simulink model "assemblage_19"  (R2016a)
settings: Solver=ode15s  StartTime=0.0  StopTime=1e6  RelTol=1e-3
undefined symbols (not defined in the file or in its folder): W
libraries: simCryogenics_lib x424, nesl_utility x343, fl_lib x9
(part 1 of 3)
settings Model: Creator=bert  LastModifiedBy=FB229602
settings DataIOCC: LimitDataPoints=on  SaveFormat=Array
settings HardwareCC: ProdBitPerPointer=32  ProdLargestAtomicFloat=None  ProdIntDivRoundTo=Undefined  ProdEndianess=Unspecified  ProdWordSize=32  ProdHWDeviceType=32-bit Generic
settings ModelReferenceCC: PropagateSignalLabelsOutOfModel=off
settings ConfigComp: CovModelRefEnable=Off
settings SimscapeCC: SimscapeLogType=all

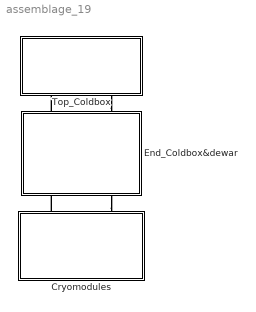
== system assemblage_19 ==
  Cryomodules : Subsystem
  End_Coldbox&dewar : Subsystem
  Top_Coldbox : Subsystem
  connections:
  End_Coldbox&dewar/RConn1 -- Top_Coldbox/LConn1
  Top_Coldbox/LConn2 -- End_Coldbox&dewar/RConn2
  End_Coldbox&dewar/LConn2 -- Cryomodules/RConn2
  Cryomodules/RConn1 -- End_Coldbox&dewar/LConn1

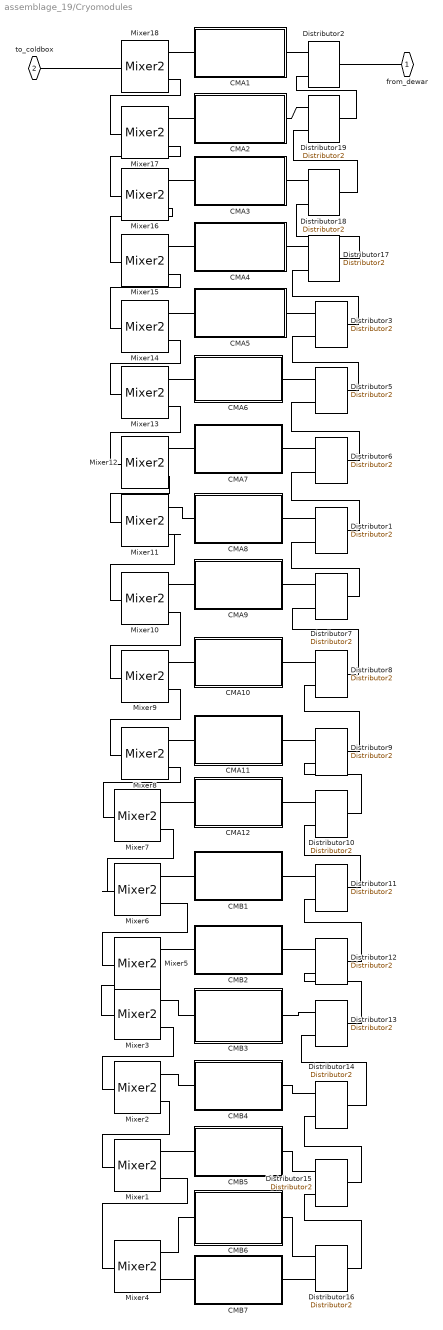
== system assemblage_19/Cryomodules ==
  CMA1 : Subsystem
  CMA10 : Subsystem
  CMA11 : Subsystem
  CMA12 : Subsystem
  CMA2 : Subsystem
  CMA3 : Subsystem
  CMA4 : Subsystem
  CMA5 : Subsystem
  CMA6 : Subsystem
  CMA7 : Subsystem
  CMA8 : Subsystem
  CMA9 : Subsystem
  CMB1 : Subsystem
  CMB2 : Subsystem
  CMB3 : Subsystem
  CMB4 : Subsystem
  CMB5 : Subsystem
  CMB6 : Subsystem
  CMB7 : Subsystem
  Distributor{1..3,5..19} (18 alike) : simCryogenics_lib/Elements/Distributor2
  Mixer{1..18} (18 alike) : simCryogenics_lib/Elements/Mixer2
  from_dewar : PMIOPort  Port=1  Side=Right
  to_coldbox : PMIOPort  Port=2  Side=Right
  connections:
  CMA1/RConn1 -- Distributor2/RConn2
  from_dewar/RConn1 -- Distributor2/LConn1
  Distributor1/RConn2 -- CMA8/RConn1
  CMA7/RConn1 -- Distributor6/RConn2
  CMA6/RConn1 -- Distributor5/RConn2
  CMA5/RConn1 -- Distributor3/RConn2
  Distributor3/RConn1 -- Distributor5/LConn1
  Distributor5/RConn1 -- Distributor6/LConn1
  Distributor6/RConn1 -- Distributor1/LConn1
  Distributor1/RConn1 -- Distributor7/LConn1
  Distributor7/RConn1 -- Distributor8/LConn1
  Distributor8/RConn1 -- Distributor9/LConn1
  Distributor10/LConn1 -- Distributor9/RConn1
  Distributor11/LConn1 -- Distributor10/RConn1
  Distributor11/RConn2 -- CMB1/RConn1
  Distributor10/RConn2 -- CMA12/RConn1
  Distributor9/RConn2 -- CMA11/RConn1
  CMA10/RConn1 -- Distributor8/RConn2
  CMA9/RConn1 -- Distributor7/RConn2
  Distributor12/LConn1 -- Distributor11/RConn1
  Distributor12/RConn2 -- CMB2/RConn1
  Distributor13/LConn1 -- Distributor12/RConn1
  Distributor13/RConn2 -- CMB3/RConn1
  Distributor14/LConn1 -- Distributor13/RConn1
  Distributor14/RConn2 -- CMB4/RConn1
  Distributor15/LConn1 -- Distributor14/RConn1
  Distributor15/RConn2 -- CMB5/RConn1
  Distributor16/LConn1 -- Distributor15/RConn1
  Distributor16/RConn2 -- CMB6/RConn1
  Distributor16/RConn1 -- CMB7/RConn1
  Distributor3/LConn1 -- Distributor17/RConn1
  Distributor17/RConn2 -- CMA4/RConn1
  Distributor18/RConn1 -- Distributor17/LConn1
  Distributor18/RConn2 -- CMA3/RConn1
  Distributor18/LConn1 -- Distributor19/RConn1
  Distributor19/RConn2 -- CMA2/RConn1
  Distributor2/RConn1 -- Distributor19/LConn1
  Mixer4/LConn1 -- CMB7/LConn1
  CMB6/LConn1 -- Mixer4/LConn2
  Mixer4/RConn1 -- Mixer1/LConn1
  CMB5/LConn1 -- Mixer1/LConn2
  Mixer2/LConn2 -- CMB4/LConn1
  Mixer1/RConn1 -- Mixer2/LConn1
  Mixer2/RConn1 -- Mixer3/LConn1
  CMB3/LConn1 -- Mixer3/LConn2
  Mixer5/LConn2 -- CMB2/LConn1
  Mixer3/RConn1 -- Mixer5/LConn1
  Mixer5/RConn1 -- Mixer6/LConn1
  Mixer6/LConn2 -- CMB1/LConn1
  Mixer6/RConn1 -- Mixer7/LConn1
  Mixer7/LConn2 -- CMA12/LConn1
  Mixer8/LConn1 -- Mixer7/RConn1
  Mixer8/LConn2 -- CMA11/LConn1
  Mixer9/LConn2 -- CMA10/LConn1
  Mixer9/LConn1 -- Mixer8/RConn1
  Mixer10/LConn2 -- CMA9/LConn1
  Mixer10/LConn1 -- Mixer9/RConn1
  Mixer11/LConn2 -- CMA8/LConn1
  Mixer11/LConn1 -- Mixer10/RConn1
  Mixer11/RConn1 -- Mixer12/LConn1
  Mixer12/LConn2 -- CMA7/LConn1
  Mixer13/LConn1 -- Mixer12/RConn1
  Mixer13/LConn2 -- CMA6/LConn1
  Mixer14/LConn1 -- Mixer13/RConn1
  Mixer14/LConn2 -- CMA5/LConn1
  Mixer15/LConn2 -- CMA4/LConn1
  Mixer15/LConn1 -- Mixer14/RConn1
  Mixer16/LConn2 -- CMA3/LConn1
  Mixer15/RConn1 -- Mixer16/LConn1
  Mixer17/LConn2 -- CMA2/LConn1
  Mixer18/LConn2 -- CMA1/LConn1
  Mixer17/LConn1 -- Mixer16/RConn1
  Mixer18/LConn1 -- Mixer17/RConn1
  Mixer18/RConn1 -- to_coldbox/RConn1

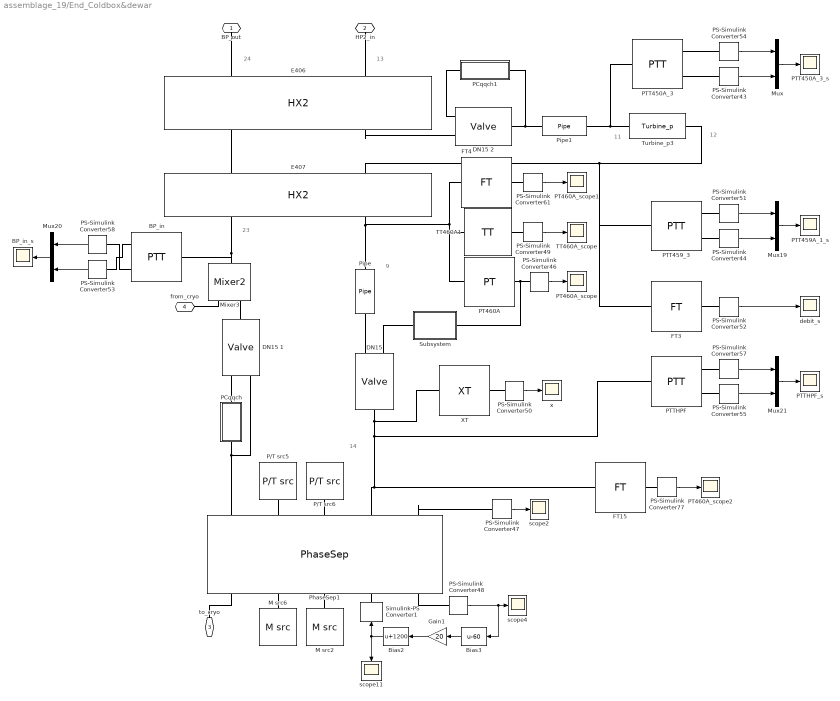
== system assemblage_19/End_Coldbox&dewar ==
  note: 13
  note: 24
  note: 9
  note: 14
  note: 11
  note: 12
  note: 23
  BP_in : simCryogenics_lib/Sensors/PTT
  "BP_in_s " : Scope
  Bias2 : Bias  Bias=1200
  Bias3 : Bias  Bias=-60
  "DN15 " : simCryogenics_lib/Elements/Valve  CVmax=1.5  ControlInputMin=0  ControlInputMax=100  Xt=0.86  Rv=10  lin_v=0  lim_v=0  K=2.4e-5 m^1.50000*kg^0.50000/s/bar^0.50000  Cmd_specify=off  Cmd_priority=High  Cmd=0  gamma_specify=off  gamma_priority=High  gamma=0  rho_specify=off  rho_priority=High  rho=0 kg/m^3  Xc_specify=off  Xc_priority=High  Xc=0  X_specify=off  X_priority=High  X=0  Y_specify=off  Y_priority=High  Y=0  CV_specify=off  CV_priority=High  CV=0
  DN15 1 : simCryogenics_lib/Elements/Valve  CVmax=40  ControlInputMin=0  ControlInputMax=100  Xt=0.86  Rv=50  lin_v=0  lim_v=0  K=2.4e-5 m^1.50000*kg^0.50000/s/bar^0.50000  Cmd_specify=off  Cmd_priority=High  Cmd=0  gamma_specify=off  gamma_priority=High  gamma=0  rho_specify=off  rho_priority=High  rho=0 kg/m^3  Xc_specify=off  Xc_priority=High  Xc=0  X_specify=off  X_priority=High  X=0  Y_specify=off  Y_priority=High  Y=0  CV_specify=off  CV_priority=High  CV=0
  DN15 2 : simCryogenics_lib/Elements/Valve  CVmax=4  ControlInputMin=0  ControlInputMax=100  Xt=0.86  Rv=50  lin_v=0  lim_v=0  K=2.4e-5 m^1.50000*kg^0.50000/s/bar^0.50000  Cmd_specify=off  Cmd_priority=High  Cmd=0  gamma_specify=off  gamma_priority=High  gamma=0  rho_specify=off  rho_priority=High  rho=0 kg/m^3  Xc_specify=off  Xc_priority=High  Xc=0  X_specify=off  X_priority=High  X=0  Y_specify=off  Y_priority=High  Y=0  CV_specify=off  CV_priority=High  CV=0
  E406 : simCryogenics_lib/Elements/HX2  N=9  Vh=0.065 m^3  Vc=0.023 m^3  M=64 kg  Kh=0.001/0.06439 s*bar/kg  Kc=0.0023/0.06368 s*bar/kg  h=1000 J/s/K  Th0=17 K  Ph0=14.73 bar  Mh0=0.06368 kg/s  Tc0=5 K  Pc0=1.05 bar  Mc0=0.06439 kg/s
  E407 : simCryogenics_lib/Elements/HX2  N=9  Vh=0.011 m^3  Vc=0.065 m^3  M=64 kg  Kh=0.002/0.06368 s*bar/kg  Kc=0.0023/0.06368 s*bar/kg  h=2000 J/s/K  Th0=5.7 K  Ph0=3.03 bar  Mh0=0.06368 kg/s  Tc0=4.4 K  Pc0=1.05 bar  Mc0=0.06368 kg/s
  FT15 : simCryogenics_lib/Sensors/FT
  FT3 : simCryogenics_lib/Sensors/FT
  FT4 : simCryogenics_lib/Sensors/FT
  Gain1 : Gain  Gain=20
  M src2 : simCryogenics_lib/Sources_Sinks/M src  M=0 kg/s
  M src6 : simCryogenics_lib/Sources_Sinks/M src  M=0 kg/s
  Mixer3 : simCryogenics_lib/Elements/Mixer2
  Mux{,19..21} (4 alike) : Mux  Inputs=2
  P/T src5 : simCryogenics_lib/Sources_Sinks/P//T src  P=5 bar  T=46.3 K
  P/T src6 : simCryogenics_lib/Sources_Sinks/P//T src  P=5 bar  T=46.3 K
  PCqqch : Subsystem
  PCqqch1 : Subsystem
  PS-Simulink Converter{43..44,46..55,57..58,61,77} (16 alike) : nesl_utility/PS-Simulink Converter  PhysicalDomain=network_engine_domain  SubClassName=ps_output  LeftPortType=input  RightPortType=output  PseudoPeriodic=off  Frequencies=[]  Unit=1  AffineConversion=off
  PT460A : simCryogenics_lib/Sensors/PT
  PT460A_scope : Scope
  PT460A_scope1 : Scope
  PT460A_scope2 : Scope
  PTT450A_3 : simCryogenics_lib/Sensors/PTT
  PTT450A_3_s : Scope
  PTT459A_1_s : Scope
  PTT459_3 : simCryogenics_lib/Sensors/PTT
  PTTHPF : simCryogenics_lib/Sensors/PTT
  PTTHPF_s : Scope
  PhaseSep1 : simCryogenics_lib/Elements/PhaseSep  Ideal1=1  DeltaT1=0.05 K  N1=10  h1=400 W/K  Ideal2=1  DeltaT2=0.05 K  N2=10  h2=400 W/K  hmax=1.601 m  S=3.4636 m^2  P0=1.3 atm  h0=20  T0=4.5 K
  Pipe : simCryogenics_lib/Elements/Pipe  Vol=0.01 m^3  Ideal=0  P0=3 bar  T0=4.6 K
  Pipe1 : simCryogenics_lib/Elements/Pipe  Vol=0.01 m^3  Ideal=0  P0=11 bar  T0=7.19 K
  Simulink-PS Converter1 : nesl_utility/Simulink-PS Converter  PhysicalDomain=network_engine_domain  SubClassName=ps_input  LeftPortType=input  RightPortType=output  PseudoPeriodic=off  Frequencies=[]  NoiseDistribution=none  NoiseParameters=[]  Unit=1  AffineConversion=off  InputFiltering=off  SimscapeFilterOrder=1  InputFilterTimeConstant=0.001  UdotUserProvided=1
  Subsystem : Subsystem
  TT460A1 : simCryogenics_lib/Sensors/TT
  TT460A_scope : Scope
  Turbine_p3 : simCryogenics_lib/Elements/Turbine_p  A=6.0851e-06 m^2  D=0.01 m  Mass=0.02 kg  cst_eff=1  eta0=0.75  Tin0=7.19 K  Pin0=14.73 bar  Pout0=3.03 bar  N0=2250 1/s  Q0=0 W  v0=0  I=0 kg*m^2  gamma_specify=off  gamma_priority=High  gamma=0  C_specify=off  C_priority=High  C=0  Z_specify=off  Z_priority=High  Z=0  Cp_specify=off  Cp_priority=High  Cp=0 kJ/kg/K  Sin_specify=off  Sin_priority=High  Sin=0 kJ/kg  T_specify=off  T_priority=High  T=0 K  HoutIs_specify=off  HoutIs_priority=High  HoutIs=0 kJ/kg  u1_specify=off  u1_priority=High  u1=0 m/s  c1_specify=off  c1_priority=High  c1=0 m/s  v_specify=off  v_priority=High  v=0  eta_specify=off  eta_priority=High  eta=0  eta_var_specify=off  eta_var_priority=High  eta_var=0  N_specify=off  N_priority=High  N=0 rad/s  Q_specify=off  Q_priority=High  Q=0 W
  XT : simCryogenics_lib/Sensors/XT
  debit_s : Scope
  scope11 : Scope
  scope2 : Scope
  scope4 : Scope
  x : Scope
  BP_out : PMIOPort  Port=1  Side=Right
  HP2_in : PMIOPort  Port=2  Side=Right
  to_cryo : PMIOPort  Port=3  Side=Left
  from_cryo : PMIOPort  Port=4  Side=Left
  wires:
  PS-Simulink Converter52/1 -> debit_s/1
  PS-Simulink Converter46/1 -> PT460A_scope/1
  PS-Simulink Converter49/1 -> TT460A_scope/1
  PS-Simulink Converter50/1 -> x/1
  PS-Simulink Converter54/1 -> Mux/1
  PS-Simulink Converter43/1 -> Mux/2
  Mux/1 -> PTT450A_3_s/1
  PS-Simulink Converter51/1 -> Mux19/1
  PS-Simulink Converter44/1 -> Mux19/2
  Mux19/1 -> PTT459A_1_s/1
  PS-Simulink Converter57/1 -> Mux21/1
  PS-Simulink Converter55/1 -> Mux21/2
  Mux21/1 -> PTTHPF_s/1
  Mux20/1 -> "BP_in_s "/1
  PS-Simulink Converter58/1 -> Mux20/1
  PS-Simulink Converter53/1 -> Mux20/2
  PS-Simulink Converter47/1 -> scope2/1
  PS-Simulink Converter61/1 -> PT460A_scope1/1
  PS-Simulink Converter77/1 -> PT460A_scope2/1
  Bias2/1 -> scope11/1, Simulink-PS Converter1/1
  PS-Simulink Converter48/1 -> Bias3/1, scope4/1
  Gain1/1 -> Bias2/1
  Bias3/1 -> Gain1/1
  connections:
  BP_in/LConn1 -- E407/RConn1 -- Mixer3/RConn1
  TT460A1/LConn1 -- PT460A/LConn1 -- FT4/LConn1 -- Pipe/LConn1 -- E407/RConn2
  E407/LConn2 -- PTT459_3/LConn1 -- FT3/LConn1 -- Turbine_p3/RConn1
  PhaseSep1/LConn4 -- FT15/LConn1 -- PTTHPF/LConn1 -- XT/LConn1 -- "DN15 "/RConn1
  PS-Simulink Converter46/LConn1 -- PT460A/RConn1 -- Subsystem/RConn1
  PhaseSep1/LConn5 -- PS-Simulink Converter47/LConn1
  BP_in/RConn1 -- PS-Simulink Converter58/LConn1
  PS-Simulink Converter50/LConn1 -- XT/RConn1
  M src2/RConn1 -- PhaseSep1/RConn3
  BP_in/RConn2 -- PS-Simulink Converter53/LConn1
  PhaseSep1/LConn2 -- P/T src5/RConn1
  E406/RConn1 -- E407/LConn1
  P/T src6/RConn1 -- PhaseSep1/LConn3
  PS-Simulink Converter44/LConn1 -- PTT459_3/RConn2
  PTT450A_3/RConn1 -- PS-Simulink Converter54/LConn1
  PS-Simulink Converter49/LConn1 -- TT460A1/RConn1
  PS-Simulink Converter55/LConn1 -- PTTHPF/RConn2
  PS-Simulink Converter52/LConn1 -- FT3/RConn1
  "DN15 "/LConn2 -- Pipe/RConn1
  M src6/RConn1 -- PhaseSep1/RConn2
  to_cryo/RConn1 -- PhaseSep1/RConn1
  PS-Simulink Converter51/LConn1 -- PTT459_3/RConn1
  PTT450A_3/RConn2 -- PS-Simulink Converter43/LConn1
  DN15 1/LConn2 -- PCqqch/LConn1 -- PhaseSep1/LConn1
  PTTHPF/RConn1 -- PS-Simulink Converter57/LConn1
  FT4/RConn1 -- PS-Simulink Converter61/LConn1
  Subsystem/LConn1 -- "DN15 "/LConn1
  FT15/RConn1 -- PS-Simulink Converter77/LConn1
  E406/LConn1 -- BP_out/RConn1
  HP2_in/RConn1 -- E406/LConn2
  PCqqch/RConn1 -- DN15 1/LConn1
  DN15 1/RConn1 -- Mixer3/LConn2
  from_cryo/RConn1 -- Mixer3/LConn1
  PCqqch1/RConn1 -- DN15 2/LConn1
  E406/RConn2 -- DN15 2/LConn2
  Turbine_p3/LConn1 -- Pipe1/RConn1 -- PTT450A_3/LConn1
  DN15 2/RConn1 -- Pipe1/LConn1 -- PCqqch1/LConn1
  PhaseSep1/RConn5 -- PS-Simulink Converter48/LConn1
  PhaseSep1/RConn4 -- Simulink-PS Converter1/RConn1

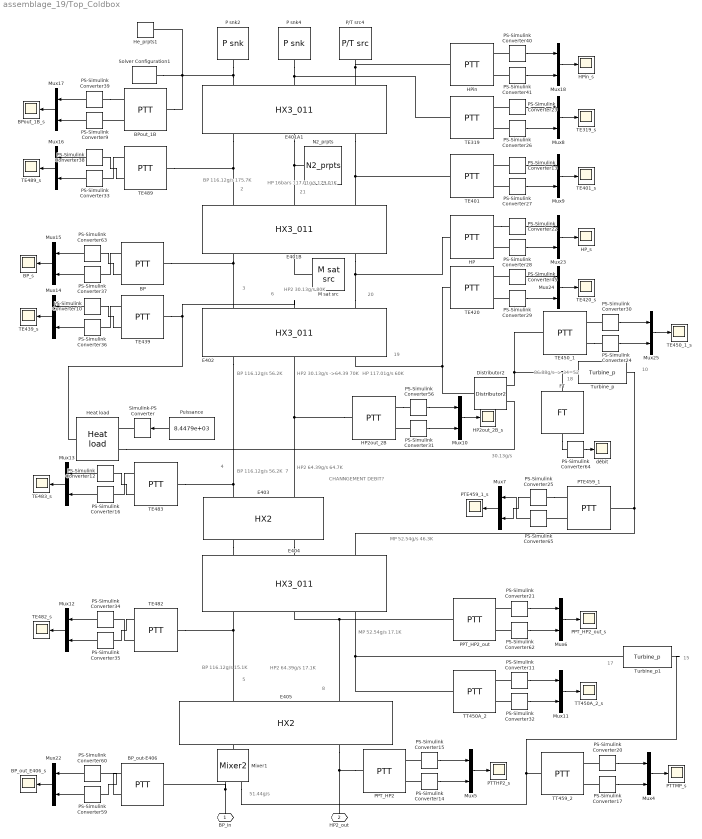
== system assemblage_19/Top_Coldbox ==
  note: 18
  note: 10
  note: 17
  note: 15
  note: 8
  note: 7
  note: 6
  note: 19
  note: 20
  note: 21
  note: 5
  note: 4
  note: 3
  note: 2
  note: HP
      | 16bars
      | 117.01g/s
      | 179.01K
  note: BP
      | 116.12g/s
      | 175.7K
  note: MP
      | 52.54g/s
      | 17.1K
  note: HP2
      | 64.39g/s
      | 17.1K
  note: BP
      | 116.12g/s
      | 15.1K
  note: MP
      | 52.54g/s
      | 46.3K
  note: CHANNGEMENT DEBIT?
  note: HP2
      | 64.39g/s
      | 64.7K
  note: BP
      | 116.12g/s
      | 56.2K
  note: 30.13g/s
  note: 86.88g/s
      | ->-34=52
  note: HP
      | 117.01g/s
      | 60K
  note: HP2
      | 30.13g/s ->64.39
      | 70K
  note: BP
      | 116.12g/s
      | 56.2K
  note: HP2
      | 30.13g/s
      | 80K
  note: 51.44g/s
  BP : simCryogenics_lib/Sensors/PTT
  BP_out-E406 : simCryogenics_lib/Sensors/PTT
  BP_out_E406_s : Scope
  BP_s : Scope
  BPout_1B : simCryogenics_lib/Sensors/PTT
  BPout_1B_s : Scope
  Distributor2 : simCryogenics_lib/Elements/Distributor2
  E401A1 : simCryogenics_lib/Elements/HX3_011  N=9  Vh=0.055 m^3  Vm=0.008 m^3  Vc=0.118 km^3  M=281 kg  Kh=0.033/0.11701 s*bar/kg  Km=0.021/.0026 s*bar/kg  Kc=0.062/0.11612 s*bar/kg  hh_m=2500 J/s/K  hh_c=1.8095e+04 J/s/K  hm_c=1 J/s/K  Th0=305 K  Ph0=14.73 bar  Mh0=0.11701 kg/s  Tm0=175.7 K  Pm0=1.1 bar  Mm0=0.0026 kg/s  Tc0=175.7 K  Pc0=1.05 bar  Mc0=0.11612 kg/s  sensh=0  sensm=1  sensc=1
  E401B : simCryogenics_lib/Elements/HX3_011  N=9  Vh=0.062 m^3  Vm=0.012 m^3  Vc=0.133 m^3  M=195 kg  Kh=0.017/0.11701 s*bar/kg  Km=0.002/(0.0026*4) s*bar/kg  Kc=0.051/0.11612 s*bar/kg  hh_m=7500 J/s/K  hh_c=25000 J/s/K  hm_c=1 J/s/K  Th0=179 K  Ph0=14.73 bar  Mh0=0.11701 kg/s  Tm0=80 K  Pm0=1.05 bar  Mm0=0.0026*4 kg/s  Tc0=80 K  Pc0=1.05 bar  Mc0=0.11612 kg/s  sensh=0  sensm=1  sensc=1
  E402 : simCryogenics_lib/Elements/HX3_011  N=9  Vh=0.133 m^3  Vm=0.005 m^3  Vc=0.012 m^3  M=195 kg  Kh=0.0255/0.11612 s*bar/kg  Km=0.011/0.03013 s*bar/kg  Kc=0.014/0.11701 s*bar/kg  hh_m=500 J/s/K  hh_c=3750 J/s/K  hm_c=1 J/s/K  Th0=56.2 K  Ph0=1.05 bar  Mh0=0.11612 kg/s  Tm0=80 K  Pm0=14.73 bar  Mm0=0.06439 kg/s  Tc0=100 K  Pc0=14.73 bar  Mc0=0.11701 kg/s  sensh=0  sensm=1  sensc=1
  E403 : simCryogenics_lib/Elements/HX2  N=9  Vh=0.049 m^3  Vc=0.172 m^3  M=227.5 kg  Kh=0.003/0.06439 s*bar/kg  Kc=0.0055/0.11612 s*bar/kg  h=5700 J/s/K  Th0=64.7 K  Ph0=14.73 bar  Mh0=0.116 kg/s  Tc0=46 K  Pc0=1.05 bar  Mc0=0.064 kg/s
  E404 : simCryogenics_lib/Elements/HX3_011  N=9  Vh=0.172 m^3  Vm=0.049 m^3  Vc=0.045 m^3  M=227.5 kg  Kh=0.0055/0.011612 s*bar/kg  Km=0.003/0.06439 s*bar/kg  Kc=0.004/0.05254 s*bar/kg  hh_m=11000 J/s/K  hh_c=8000 J/s/K  hm_c=1 J/s/K  Th0=15.1 K  Ph0=1.05 bar  Mh0=0.116 kg/s  Tm0=46 K  Pm0=14.73 bar  Mm0=0.064 kg/s  Tc0=46.3 K  Pc0=5 bar  Mc0=0.052 kg/s  sensh=0  sensm=1  sensc=1
  "E405 " : simCryogenics_lib/Elements/HX2  N=9  Vh=0.023 m^3  Vc=0.065 m^3  M=64 kg  Kh=0.001/0.6439 s*bar/kg  Kc=0.0023/0.11612 s*bar/kg  h=1500 J/s/K  Th0=17.1 K  Ph0=14.73 bar  Mh0=0.11612 kg/s  Tc0=10 K  Pc0=1.05 bar  Mc0=0.06439 kg/s
  FT : simCryogenics_lib/Sensors/FT
  HP : simCryogenics_lib/Sensors/PTT
  HP2out_2B : simCryogenics_lib/Sensors/PTT
  HP2out_2B_s : Scope
  HP_s : Scope
  HPin : simCryogenics_lib/Sensors/PTT
  HPin_s : Scope
  He_prpts1 : simCryogenics_lib/Utilities/He_prpts  P_min=0.1 bar  P_max=30 bar  T_min=3 K  T_max=320 K  N=100  Mol=4.0026 * 10 ^ (- 3) kg/mol
  Heat load : simCryogenics_lib/Utilities/Heat load
  M sat src : simCryogenics_lib/Sources_Sinks/M sat src  M=0.015 kg/s  Xmix=0
  Mixer1 : simCryogenics_lib/Elements/Mixer2
  Mux{4..18,22..25} (19 alike) : Mux  Inputs=2
  N2_prpts : simCryogenics_lib/Utilities/N2_prpts  P_min=0.5 bar  T_min=70 K  T_max=320 K  P_max=20 bar  Mol=4.0026 * (10 ^ (- 3)) kg/mol
  P snk2 : simCryogenics_lib/Sources_Sinks/P snk  P=1.05 bar
  P snk4 : simCryogenics_lib/Sources_Sinks/P snk  P=1.05 bar
  P/T src4 : simCryogenics_lib/Sources_Sinks/P//T src  P=14.73 bar  T=305 K
  PPT_HP2 : simCryogenics_lib/Sensors/PTT
  PPT_HP2_out : simCryogenics_lib/Sensors/PTT
  PPT_HP2_out_s : Scope
  PS-Simulink Converter{9..17,20..41,45,56,59..60,62..65} (39 alike) : nesl_utility/PS-Simulink Converter  PhysicalDomain=network_engine_domain  SubClassName=ps_output  LeftPortType=input  RightPortType=output  PseudoPeriodic=off  Frequencies=[]  Unit=1  AffineConversion=off
  PTE459_1 : simCryogenics_lib/Sensors/PTT
  PTE459_1_s : Scope
  PTTHP2_s : Scope
  PTTMP_s : Scope
  "Puissance " : Constant  Value=8.4479e+03
  Simulink-PS Converter : nesl_utility/Simulink-PS Converter  PhysicalDomain=network_engine_domain  SubClassName=ps_input  LeftPortType=input  RightPortType=output  PseudoPeriodic=off  Frequencies=[]  NoiseDistribution=none  NoiseParameters=[]  Unit=1  AffineConversion=off  InputFiltering=off  SimscapeFilterOrder=1  InputFilterTimeConstant=0.001  UdotUserProvided=1
  Solver Configuration1 : nesl_utility/Solver Configuration  PhysicalDomain=network_engine_domain  SubClassName=solver  LeftPortType=input  RightPortType=generic  Accelerate=off  Tones=[]  Harmonics=[]  SimulateNoise=off  Profile=off  UseLocalSampling=off  EnableSwitchedLinearOptims=on  FrequencyDomain=off  UseCCode=off  RelTol=0.001  AbsTol=1e-06  MinStep=1e-09  ToWorkspace=off  RevertToSquareIcSolve=off  NumHomotopyIterations=100  PhasorMode=off  PhasorModeNumHarmonics=1  OverrideAbsTol=off  DoDC=off  ResidualTolerance=1e-09  UseLocalSolver=off  LocalSolverChoice=NE_BACKWARD_EULER_ADVANCER  LocalSolverSampleTime=0.001  DoFixedCost=off  MaxNonlinIter=3  MaxModeIter=2  LinearAlgebra=Sparse  DelaysMemoryBudget=1024  AutomaticFiltering=on  FilteringTimeConstant=0.001
  TE{319,401,420,439,482..483,489} (7 alike) : simCryogenics_lib/Sensors/PTT
  TE319_s : Scope
  TE401_s : Scope
  TE420_s : Scope
  TE439_s : Scope
  TE450_1 : simCryogenics_lib/Sensors/PTT
  TE450_1_s : Scope
  TE482_s : Scope
  TE483_s : Scope
  TE489_s : Scope
  TT450A_2 : simCryogenics_lib/Sensors/PTT
  TT450A_2_s : Scope
  TT459_2 : simCryogenics_lib/Sensors/PTT
  Turbine_p : simCryogenics_lib/Elements/Turbine_p  A=1.7590e-05 m^2  D=0.035 m  Mass=0.02 kg  cst_eff=1  eta0=0.75  Tin0=80 K  Pin0=14.73 bar  Pout0=5.3 bar  N0=2250 1/s  Q0=0 W  v0=0  I=0 kg*m^2  gamma_specify=off  gamma_priority=High  gamma=0  C_specify=off  C_priority=High  C=0  Z_specify=off  Z_priority=High  Z=0  Cp_specify=off  Cp_priority=High  Cp=0 kJ/kg/K  Sin_specify=off  Sin_priority=High  Sin=0 kJ/kg  T_specify=off  T_priority=High  T=0 K  HoutIs_specify=off  HoutIs_priority=High  HoutIs=0 kJ/kg  u1_specify=off  u1_priority=High  u1=0 m/s  c1_specify=off  c1_priority=High  c1=0 m/s  v_specify=off  v_priority=High  v=0  eta_specify=off  eta_priority=High  eta=0  eta_var_specify=off  eta_var_priority=High  eta_var=0  N_specify=off  N_priority=High  N=0 rad/s  Q_specify=off  Q_priority=High  Q=0 W
  Turbine_p1 : simCryogenics_lib/Elements/Turbine_p  A=2.6523e-05 m^2  D=0.02 m  Mass=0.02 kg  cst_eff=1  eta0=0.75  Tin0=17.1 K  Pin0=5 bar  Pout0=1.3 bar  N0=2250 1/s  Q0=0 W  v0=0  I=0 kg*m^2  gamma_specify=off  gamma_priority=High  gamma=0  C_specify=off  C_priority=High  C=0  Z_specify=off  Z_priority=High  Z=0  Cp_specify=off  Cp_priority=High  Cp=0 kJ/kg/K  Sin_specify=off  Sin_priority=High  Sin=0 kJ/kg  T_specify=off  T_priority=High  T=0 K  HoutIs_specify=off  HoutIs_priority=High  HoutIs=0 kJ/kg  u1_specify=off  u1_priority=High  u1=0 m/s  c1_specify=off  c1_priority=High  c1=0 m/s  v_specify=off  v_priority=High  v=0  eta_specify=off  eta_priority=High  eta=0  eta_var_specify=off  eta_var_priority=High  eta_var=0  N_specify=off  N_priority=High  N=0 rad/s  Q_specify=off  Q_priority=High  Q=0 W
  débit : Scope
  BP_in : PMIOPort  Port=1  Side=Left
  HP2_out : PMIOPort  Port=2  Side=Left
  wires:
  "Puissance "/1 -> Simulink-PS Converter/1
  PS-Simulink Converter64/1 -> débit/1
  PS-Simulink Converter15/1 -> Mux5/1
  PS-Simulink Converter14/1 -> Mux5/2
  Mux5/1 -> PTTHP2_s/1
  PS-Simulink Converter20/1 -> Mux4/1
  PS-Simulink Converter17/1 -> Mux4/2
  Mux4/1 -> PTTMP_s/1
  PS-Simulink Converter21/1 -> Mux6/1
  PS-Simulink Converter62/1 -> Mux6/2
  Mux6/1 -> PPT_HP2_out_s/1
  Mux7/1 -> PTE459_1_s/1
  PS-Simulink Converter23/1 -> Mux8/1
  PS-Simulink Converter26/1 -> Mux8/2
  Mux8/1 -> TE319_s/1
  PS-Simulink Converter13/1 -> Mux9/1
  PS-Simulink Converter27/1 -> Mux9/2
  Mux9/1 -> TE401_s/1
  PS-Simulink Converter28/1 -> Mux23/2
  Mux23/1 -> HP_s/1
  PS-Simulink Converter45/1 -> Mux24/1
  PS-Simulink Converter29/1 -> Mux24/2
  Mux24/1 -> TE420_s/1
  PS-Simulink Converter30/1 -> Mux25/1
  Mux25/1 -> TE450_1_s/1
  PS-Simulink Converter22/1 -> Mux23/1
  PS-Simulink Converter31/1 -> Mux10/2
  Mux10/1 -> HP2out_2B_s/1
  PS-Simulink Converter56/1 -> Mux10/1
  PS-Simulink Converter11/1 -> Mux11/1
  PS-Simulink Converter32/1 -> Mux11/2
  Mux11/1 -> TT450A_2_s/1
  Mux12/1 -> TE482_s/1
  PS-Simulink Converter34/1 -> Mux12/1
  PS-Simulink Converter35/1 -> Mux12/2
  Mux13/1 -> TE483_s/1
  PS-Simulink Converter12/1 -> Mux13/1
  PS-Simulink Converter16/1 -> Mux13/2
  Mux14/1 -> TE439_s/1
  PS-Simulink Converter10/1 -> Mux14/1
  PS-Simulink Converter36/1 -> Mux14/2
  Mux15/1 -> BP_s/1
  PS-Simulink Converter63/1 -> Mux15/1
  PS-Simulink Converter37/1 -> Mux15/2
  Mux16/1 -> TE489_s/1
  PS-Simulink Converter38/1 -> Mux16/1
  PS-Simulink Converter33/1 -> Mux16/2
  Mux17/1 -> BPout_1B_s/1
  PS-Simulink Converter39/1 -> Mux17/1
  PS-Simulink Converter9/1 -> Mux17/2
  PS-Simulink Converter65/1 -> Mux7/1
  PS-Simulink Converter25/1 -> Mux7/2
  PS-Simulink Converter24/1 -> Mux25/2
  PS-Simulink Converter40/1 -> Mux18/1
  PS-Simulink Converter41/1 -> Mux18/2
  Mux18/1 -> HPin_s/1
  Mux22/1 -> BP_out_E406_s/1
  PS-Simulink Converter60/1 -> Mux22/1
  PS-Simulink Converter59/1 -> Mux22/2
  connections:
  TE482/LConn1 -- "E405 "/LConn1 -- E404/LConn3
  TE483/LConn1 -- E402/LConn3 -- E403/LConn1
  HP2out_2B/LConn1 -- E403/LConn2 -- E402/LConn2
  PPT_HP2_out/LConn1 -- "E405 "/LConn2 -- E404/LConn2
  Turbine_p1/LConn1 -- TT450A_2/LConn1 -- E404/LConn1
  PTE459_1/LConn1 -- Turbine_p/RConn1 -- E404/RConn1
  BP/LConn1 -- E401B/RConn1 -- E402/RConn3
  E401A1/RConn1 -- TE489/LConn1 -- E401B/LConn1
  E402/RConn1 -- HP/LConn1 -- E401B/RConn3
  E402/LConn1 -- Distributor2/LConn1 -- TE420/LConn1
  E402/RConn2 -- Heat load/RConn1 -- TE439/LConn1
  Turbine_p/LConn1 -- FT/LConn1 -- TE450_1/LConn1 -- Distributor2/RConn1
  Turbine_p1/RConn1 -- Mixer1/LConn2 -- TT459_2/LConn1
  E401A1/RConn3 -- E401B/LConn3 -- TE401/LConn1
  PPT_HP2/LConn1 -- "E405 "/RConn2 -- HP2_out/RConn1
  Mixer1/LConn1 -- BP_in/RConn1 -- BP_out-E406/LConn1
  HPin/LConn1 -- P/T src4/RConn1 -- E401A1/LConn3
  E401A1/LConn2 -- P snk4/RConn1 -- TE319/LConn1
  E401A1/LConn1 -- Solver Configuration1/RConn1 -- He_prpts1/RConn1 -- BPout_1B/LConn1 -- P snk2/RConn1
  PS-Simulink Converter38/LConn1 -- TE489/RConn1
  TE489/RConn2 -- PS-Simulink Converter33/LConn1
  BPout_1B/RConn2 -- PS-Simulink Converter9/LConn1
  PS-Simulink Converter39/LConn1 -- BPout_1B/RConn1
  PS-Simulink Converter40/LConn1 -- HPin/RConn1
  PS-Simulink Converter41/LConn1 -- HPin/RConn2
  BP_out-E406/RConn1 -- PS-Simulink Converter60/LConn1
  PS-Simulink Converter26/LConn1 -- TE319/RConn2
  E403/RConn2 -- E404/RConn2
  PS-Simulink Converter25/LConn1 -- PTE459_1/RConn2
  TE450_1/RConn2 -- PS-Simulink Converter24/LConn1
  PS-Simulink Converter62/LConn1 -- PPT_HP2_out/RConn2
  PS-Simulink Converter11/LConn1 -- TT450A_2/RConn1
  PS-Simulink Converter21/LConn1 -- PPT_HP2_out/RConn1
  PS-Simulink Converter20/LConn1 -- TT459_2/RConn1
  PS-Simulink Converter32/LConn1 -- TT450A_2/RConn2
  E401A1/RConn2 -- N2_prpts/RConn1 -- E401B/LConn2
  M sat src/RConn1 -- E401B/RConn2
  PS-Simulink Converter17/LConn1 -- TT459_2/RConn2
  PS-Simulink Converter31/LConn1 -- HP2out_2B/RConn2
  PS-Simulink Converter15/LConn1 -- PPT_HP2/RConn1
  HP2out_2B/RConn1 -- PS-Simulink Converter56/LConn1
  PS-Simulink Converter14/LConn1 -- PPT_HP2/RConn2
  Mixer1/RConn1 -- "E405 "/RConn1
  HP/RConn1 -- PS-Simulink Converter22/LConn1
  FT/RConn1 -- PS-Simulink Converter64/LConn1
  PS-Simulink Converter30/LConn1 -- TE450_1/RConn1
  PS-Simulink Converter29/LConn1 -- TE420/RConn2
  PS-Simulink Converter45/LConn1 -- TE420/RConn1
  Simulink-PS Converter/RConn1 -- Heat load/LConn2
  Heat load/LConn1 -- Distributor2/RConn2
  PS-Simulink Converter28/LConn1 -- HP/RConn2
  PS-Simulink Converter13/LConn1 -- TE401/RConn1
  PS-Simulink Converter27/LConn1 -- TE401/RConn2
  PTE459_1/RConn1 -- PS-Simulink Converter65/LConn1
  E403/RConn1 -- E404/RConn3
  BP_out-E406/RConn2 -- PS-Simulink Converter59/LConn1
  PS-Simulink Converter23/LConn1 -- TE319/RConn1
  TE483/RConn2 -- PS-Simulink Converter16/LConn1
  PS-Simulink Converter12/LConn1 -- TE483/RConn1
  TE482/RConn2 -- PS-Simulink Converter35/LConn1
  TE482/RConn1 -- PS-Simulink Converter34/LConn1
  TE439/RConn2 -- PS-Simulink Converter36/LConn1
  PS-Simulink Converter10/LConn1 -- TE439/RConn1
  BP/RConn2 -- PS-Simulink Converter37/LConn1
  PS-Simulink Converter63/LConn1 -- BP/RConn1

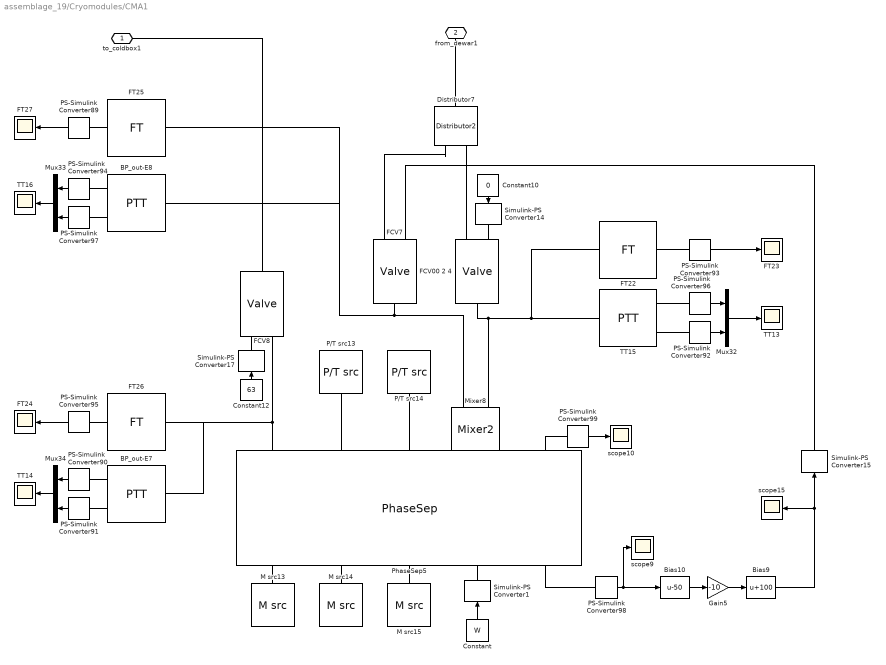
== system assemblage_19/Cryomodules/CMA1 ==
  BP_out-E7 : simCryogenics_lib/Sensors/PTT
  BP_out-E8 : simCryogenics_lib/Sensors/PTT
  Bias10 : Bias  Bias=-50
  Bias9 : Bias  Bias=100
  Constant : Constant  Value=W
  Constant10 : Constant  Value=0
  Constant12 : Constant  Value=63
  Distributor7 : simCryogenics_lib/Elements/Distributor2
  FCV00 2 4 : simCryogenics_lib/Elements/Valve  CVmax=0.2  ControlInputMin=0  ControlInputMax=100  Xt=0.86  Rv=100  lin_v=0  lim_v=0  K=2.4e-5 m^1.50000*kg^0.50000/s/bar^0.50000  Cmd_specify=off  Cmd_priority=High  Cmd=0  gamma_specify=off  gamma_priority=High  gamma=0  rho_specify=off  rho_priority=High  rho=0 kg/m^3  Xc_specify=off  Xc_priority=High  Xc=0  X_specify=off  X_priority=High  X=0  Y_specify=off  Y_priority=High  Y=0  CV_specify=off  CV_priority=High  CV=0
  FCV7 : simCryogenics_lib/Elements/Valve  CVmax=1.25  ControlInputMin=0  ControlInputMax=100  Xt=0.86  Rv=150  lin_v=0  lim_v=0  K=2.4e-5 m^1.50000*kg^0.50000/s/bar^0.50000  Cmd_specify=off  Cmd_priority=High  Cmd=0  gamma_specify=off  gamma_priority=High  gamma=0  rho_specify=off  rho_priority=High  rho=0 kg/m^3  Xc_specify=off  Xc_priority=High  Xc=0  X_specify=off  X_priority=High  X=0  Y_specify=off  Y_priority=High  Y=0  CV_specify=off  CV_priority=High  CV=0
  FCV8 : simCryogenics_lib/Elements/Valve  CVmax=1.5  ControlInputMin=0  ControlInputMax=100  Xt=0.86  Rv=100  lin_v=0  lim_v=0  K=2.4e-5 m^1.50000*kg^0.50000/s/bar^0.50000  Cmd_specify=off  Cmd_priority=High  Cmd=0  gamma_specify=off  gamma_priority=High  gamma=0  rho_specify=off  rho_priority=High  rho=0 kg/m^3  Xc_specify=off  Xc_priority=High  Xc=0  X_specify=off  X_priority=High  X=0  Y_specify=off  Y_priority=High  Y=0  CV_specify=off  CV_priority=High  CV=0
  FT22 : simCryogenics_lib/Sensors/FT
  FT23 : Scope
  FT24 : Scope
  FT25 : simCryogenics_lib/Sensors/FT
  FT26 : simCryogenics_lib/Sensors/FT
  FT27 : Scope
  Gain5 : Gain  Gain=-10
  M src13 : simCryogenics_lib/Sources_Sinks/M src  M=0 kg/s
  M src14 : simCryogenics_lib/Sources_Sinks/M src  M=0 kg/s
  M src15 : simCryogenics_lib/Sources_Sinks/M src  M=0 kg/s
  Mixer8 : simCryogenics_lib/Elements/Mixer2
  Mux32 : Mux  Inputs=2
  Mux33 : Mux  Inputs=2
  Mux34 : Mux  Inputs=2
  P/T src13 : simCryogenics_lib/Sources_Sinks/P//T src  P=1.2 bar  T=4.4 K
  P/T src14 : simCryogenics_lib/Sources_Sinks/P//T src  P=1.2 bar  T=4.4 K
  PS-Simulink Converter{89..99} (11 alike) : nesl_utility/PS-Simulink Converter  PhysicalDomain=network_engine_domain  SubClassName=ps_output  LeftPortType=input  RightPortType=output  PseudoPeriodic=off  Frequencies=[]  Unit=1  AffineConversion=off
  PhaseSep5 : simCryogenics_lib/Elements/PhaseSep  Ideal1=1  DeltaT1=0.05 K  N1=10  h1=400 W/K  Ideal2=1  DeltaT2=0.05 K  N2=10  h2=400 W/K  hmax=0.870 m  S=0.0402 m^2  P0=1.25 bar  h0=50  T0=4.5 K
  Simulink-PS Converter{1,14..15,17} (4 alike) : nesl_utility/Simulink-PS Converter  PhysicalDomain=network_engine_domain  SubClassName=ps_input  LeftPortType=input  RightPortType=output  PseudoPeriodic=off  Frequencies=[]  NoiseDistribution=none  NoiseParameters=[]  Unit=1  AffineConversion=off  InputFiltering=off  SimscapeFilterOrder=1  InputFilterTimeConstant=0.001  UdotUserProvided=1
  TT13 : Scope
  TT14 : Scope
  TT15 : simCryogenics_lib/Sensors/PTT
  TT16 : Scope
  scope10 : Scope
  scope15 : Scope
  scope9 : Scope
  to_coldbox1 : PMIOPort  Port=1  Side=Left
  from_dewar1 : PMIOPort  Port=2  Side=Right
  wires:
  Constant10/1 -> Simulink-PS Converter14/1
  PS-Simulink Converter99/1 -> scope10/1
  PS-Simulink Converter90/1 -> Mux34/1
  PS-Simulink Converter95/1 -> FT24/1
  Bias10/1 -> Gain5/1
  PS-Simulink Converter96/1 -> Mux32/1
  Constant/1 -> Simulink-PS Converter1/1
  Bias9/1 -> scope15/1, Simulink-PS Converter15/1
  Mux33/1 -> TT16/1
  PS-Simulink Converter89/1 -> FT27/1
  PS-Simulink Converter97/1 -> Mux33/2
  PS-Simulink Converter94/1 -> Mux33/1
  PS-Simulink Converter91/1 -> Mux34/2
  PS-Simulink Converter93/1 -> FT23/1
  Mux34/1 -> TT14/1
  PS-Simulink Converter92/1 -> Mux32/2
  Gain5/1 -> Bias9/1
  PS-Simulink Converter98/1 -> scope9/1, Bias10/1
  Mux32/1 -> TT13/1
  Constant12/1 -> Simulink-PS Converter17/1
  connections:
  BP_out-E8/RConn1 -- PS-Simulink Converter97/LConn1
  Simulink-PS Converter14/RConn1 -- FCV00 2 4/LConn1
  Distributor7/RConn2 -- FCV7/LConn2
  PS-Simulink Converter98/LConn1 -- PhaseSep5/RConn5
  from_dewar1/RConn1 -- Distributor7/LConn1
  TT15/RConn1 -- PS-Simulink Converter96/LConn1
  PhaseSep5/LConn2 -- P/T src13/RConn1
  FCV8/LConn2 -- PhaseSep5/LConn1 -- BP_out-E7/LConn1 -- FT26/LConn1
  FCV8/RConn1 -- to_coldbox1/RConn1
  P/T src14/RConn1 -- PhaseSep5/LConn3
  BP_out-E7/RConn2 -- PS-Simulink Converter90/LConn1
  FT22/LConn1 -- TT15/LConn1 -- FCV00 2 4/RConn1 -- Mixer8/LConn1
  FCV7/RConn1 -- Mixer8/LConn2 -- FT25/LConn1 -- BP_out-E8/LConn1
  Simulink-PS Converter15/RConn1 -- FCV7/LConn1
  M src15/RConn1 -- PhaseSep5/RConn3
  Simulink-PS Converter1/RConn1 -- PhaseSep5/RConn4
  BP_out-E7/RConn1 -- PS-Simulink Converter91/LConn1
  PS-Simulink Converter93/LConn1 -- FT22/RConn1
  BP_out-E8/RConn2 -- PS-Simulink Converter94/LConn1
  PhaseSep5/RConn2 -- M src14/RConn1
  PS-Simulink Converter89/LConn1 -- FT25/RConn1
  PS-Simulink Converter99/LConn1 -- PhaseSep5/LConn5
  TT15/RConn2 -- PS-Simulink Converter92/LConn1
  FCV00 2 4/LConn2 -- Distributor7/RConn1
  M src13/RConn1 -- PhaseSep5/RConn1
  PS-Simulink Converter95/LConn1 -- FT26/RConn1
  FCV8/LConn1 -- Simulink-PS Converter17/RConn1
  PhaseSep5/LConn4 -- Mixer8/RConn1

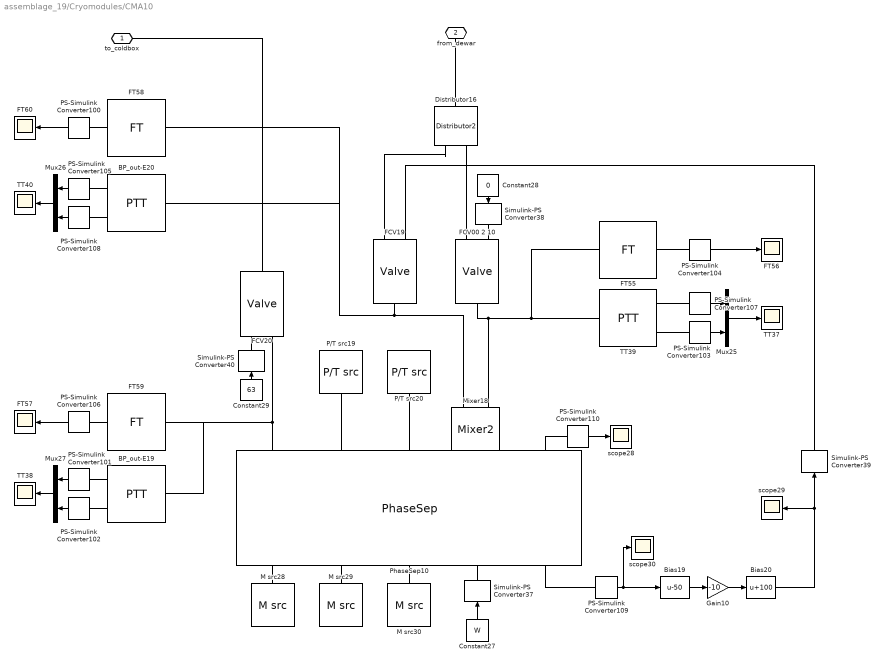
== system assemblage_19/Cryomodules/CMA10 ==
  BP_out-E19 : simCryogenics_lib/Sensors/PTT
  BP_out-E20 : simCryogenics_lib/Sensors/PTT
  Bias19 : Bias  Bias=-50
  Bias20 : Bias  Bias=100
  Constant27 : Constant  Value=W
  Constant28 : Constant  Value=0
  Constant29 : Constant  Value=63
  Distributor16 : simCryogenics_lib/Elements/Distributor2
  FCV00 2 10 : simCryogenics_lib/Elements/Valve  CVmax=0.2  ControlInputMin=0  ControlInputMax=100  Xt=0.86  Rv=100  lin_v=0  lim_v=0  K=2.4e-5 m^1.50000*kg^0.50000/s/bar^0.50000  Cmd_specify=off  Cmd_priority=High  Cmd=0  gamma_specify=off  gamma_priority=High  gamma=0  rho_specify=off  rho_priority=High  rho=0 kg/m^3  Xc_specify=off  Xc_priority=High  Xc=0  X_specify=off  X_priority=High  X=0  Y_specify=off  Y_priority=High  Y=0  CV_specify=off  CV_priority=High  CV=0
  FCV19 : simCryogenics_lib/Elements/Valve  CVmax=1.25  ControlInputMin=0  ControlInputMax=100  Xt=0.86  Rv=150  lin_v=0  lim_v=0  K=2.4e-5 m^1.50000*kg^0.50000/s/bar^0.50000  Cmd_specify=off  Cmd_priority=High  Cmd=0  gamma_specify=off  gamma_priority=High  gamma=0  rho_specify=off  rho_priority=High  rho=0 kg/m^3  Xc_specify=off  Xc_priority=High  Xc=0  X_specify=off  X_priority=High  X=0  Y_specify=off  Y_priority=High  Y=0  CV_specify=off  CV_priority=High  CV=0
  FCV20 : simCryogenics_lib/Elements/Valve  CVmax=1.5  ControlInputMin=0  ControlInputMax=100  Xt=0.86  Rv=100  lin_v=0  lim_v=0  K=2.4e-5 m^1.50000*kg^0.50000/s/bar^0.50000  Cmd_specify=off  Cmd_priority=High  Cmd=0  gamma_specify=off  gamma_priority=High  gamma=0  rho_specify=off  rho_priority=High  rho=0 kg/m^3  Xc_specify=off  Xc_priority=High  Xc=0  X_specify=off  X_priority=High  X=0  Y_specify=off  Y_priority=High  Y=0  CV_specify=off  CV_priority=High  CV=0
  FT55 : simCryogenics_lib/Sensors/FT
  FT56 : Scope
  FT57 : Scope
  FT58 : simCryogenics_lib/Sensors/FT
  FT59 : simCryogenics_lib/Sensors/FT
  FT60 : Scope
  Gain10 : Gain  Gain=-10
  M src28 : simCryogenics_lib/Sources_Sinks/M src  M=0 kg/s
  M src29 : simCryogenics_lib/Sources_Sinks/M src  M=0 kg/s
  M src30 : simCryogenics_lib/Sources_Sinks/M src  M=0 kg/s
  Mixer18 : simCryogenics_lib/Elements/Mixer2
  Mux25 : Mux  Inputs=2
  Mux26 : Mux  Inputs=2
  Mux27 : Mux  Inputs=2
  P/T src19 : simCryogenics_lib/Sources_Sinks/P//T src  P=1.2 bar  T=4.4 K
  P/T src20 : simCryogenics_lib/Sources_Sinks/P//T src  P=1.2 bar  T=4.4 K
  PS-Simulink Converter{100..110} (11 alike) : nesl_utility/PS-Simulink Converter  PhysicalDomain=network_engine_domain  SubClassName=ps_output  LeftPortType=input  RightPortType=output  PseudoPeriodic=off  Frequencies=[]  Unit=1  AffineConversion=off
  PhaseSep10 : simCryogenics_lib/Elements/PhaseSep  Ideal1=1  DeltaT1=0.05 K  N1=10  h1=400 W/K  Ideal2=1  DeltaT2=0.05 K  N2=10  h2=400 W/K  hmax=0.870 m  S=0.0402 m^2  P0=1.25 bar  h0=50  T0=4.5 K
  Simulink-PS Converter{37..40} (4 alike) : nesl_utility/Simulink-PS Converter  PhysicalDomain=network_engine_domain  SubClassName=ps_input  LeftPortType=input  RightPortType=output  PseudoPeriodic=off  Frequencies=[]  NoiseDistribution=none  NoiseParameters=[]  Unit=1  AffineConversion=off  InputFiltering=off  SimscapeFilterOrder=1  InputFilterTimeConstant=0.001  UdotUserProvided=1
  TT37 : Scope
  TT38 : Scope
  TT39 : simCryogenics_lib/Sensors/PTT
  TT40 : Scope
  scope28 : Scope
  scope29 : Scope
  scope30 : Scope
  to_coldbox : PMIOPort  Port=1  Side=Left
  from_dewar : PMIOPort  Port=2  Side=Right
  wires:
  PS-Simulink Converter109/1 -> scope30/1, Bias19/1
  PS-Simulink Converter106/1 -> FT57/1
  Constant29/1 -> Simulink-PS Converter40/1
  PS-Simulink Converter107/1 -> Mux25/1
  Mux26/1 -> TT40/1
  PS-Simulink Converter100/1 -> FT60/1
  PS-Simulink Converter101/1 -> Mux27/1
  PS-Simulink Converter110/1 -> scope28/1
  PS-Simulink Converter104/1 -> FT56/1
  Bias19/1 -> Gain10/1
  Constant28/1 -> Simulink-PS Converter38/1
  Mux25/1 -> TT37/1
  Gain10/1 -> Bias20/1
  Bias20/1 -> scope29/1, Simulink-PS Converter39/1
  Constant27/1 -> Simulink-PS Converter37/1
  PS-Simulink Converter105/1 -> Mux26/1
  PS-Simulink Converter108/1 -> Mux26/2
  PS-Simulink Converter102/1 -> Mux27/2
  Mux27/1 -> TT38/1
  PS-Simulink Converter103/1 -> Mux25/2
  connections:
  PhaseSep10/RConn2 -- M src29/RConn1
  TT39/RConn1 -- PS-Simulink Converter107/LConn1
  FT55/LConn1 -- TT39/LConn1 -- FCV00 2 10/RConn1 -- Mixer18/LConn1
  Distributor16/RConn2 -- FCV19/LConn2
  FCV20/LConn1 -- Simulink-PS Converter40/RConn1
  FCV19/RConn1 -- Mixer18/LConn2 -- FT58/LConn1 -- BP_out-E20/LConn1
  FCV00 2 10/LConn2 -- Distributor16/RConn1
  P/T src20/RConn1 -- PhaseSep10/LConn3
  Simulink-PS Converter39/RConn1 -- FCV19/LConn1
  PS-Simulink Converter106/LConn1 -- FT59/RConn1
  TT39/RConn2 -- PS-Simulink Converter103/LConn1
  PS-Simulink Converter104/LConn1 -- FT55/RConn1
  BP_out-E19/RConn1 -- PS-Simulink Converter102/LConn1
  PS-Simulink Converter110/LConn1 -- PhaseSep10/LConn5
  PhaseSep10/LConn4 -- Mixer18/RConn1
  PhaseSep10/LConn2 -- P/T src19/RConn1
  BP_out-E20/RConn1 -- PS-Simulink Converter108/LConn1
  from_dewar/RConn1 -- Distributor16/LConn1
  Simulink-PS Converter37/RConn1 -- PhaseSep10/RConn4
  FCV20/RConn1 -- to_coldbox/RConn1
  Simulink-PS Converter38/RConn1 -- FCV00 2 10/LConn1
  PS-Simulink Converter109/LConn1 -- PhaseSep10/RConn5
  BP_out-E19/RConn2 -- PS-Simulink Converter101/LConn1
  M src28/RConn1 -- PhaseSep10/RConn1
  M src30/RConn1 -- PhaseSep10/RConn3
  FCV20/LConn2 -- PhaseSep10/LConn1 -- BP_out-E19/LConn1 -- FT59/LConn1
  BP_out-E20/RConn2 -- PS-Simulink Converter105/LConn1
  PS-Simulink Converter100/LConn1 -- FT58/RConn1

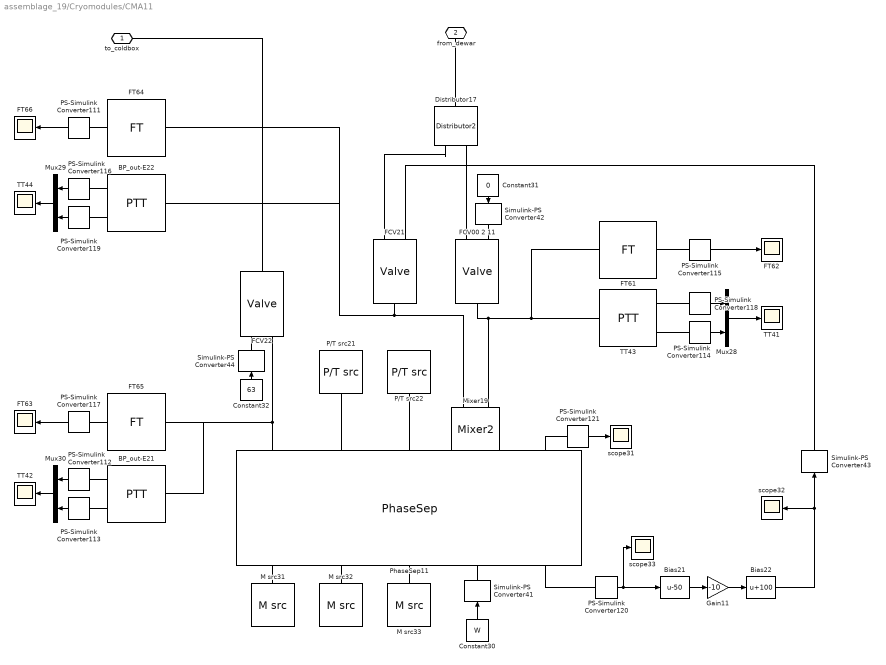
== system assemblage_19/Cryomodules/CMA11 ==
  BP_out-E21 : simCryogenics_lib/Sensors/PTT
  BP_out-E22 : simCryogenics_lib/Sensors/PTT
  Bias21 : Bias  Bias=-50
  Bias22 : Bias  Bias=100
  Constant30 : Constant  Value=W
  Constant31 : Constant  Value=0
  Constant32 : Constant  Value=63
  Distributor17 : simCryogenics_lib/Elements/Distributor2
  FCV00 2 11 : simCryogenics_lib/Elements/Valve  CVmax=0.2  ControlInputMin=0  ControlInputMax=100  Xt=0.86  Rv=100  lin_v=0  lim_v=0  K=2.4e-5 m^1.50000*kg^0.50000/s/bar^0.50000  Cmd_specify=off  Cmd_priority=High  Cmd=0  gamma_specify=off  gamma_priority=High  gamma=0  rho_specify=off  rho_priority=High  rho=0 kg/m^3  Xc_specify=off  Xc_priority=High  Xc=0  X_specify=off  X_priority=High  X=0  Y_specify=off  Y_priority=High  Y=0  CV_specify=off  CV_priority=High  CV=0
  FCV21 : simCryogenics_lib/Elements/Valve  CVmax=1.25  ControlInputMin=0  ControlInputMax=100  Xt=0.86  Rv=150  lin_v=0  lim_v=0  K=2.4e-5 m^1.50000*kg^0.50000/s/bar^0.50000  Cmd_specify=off  Cmd_priority=High  Cmd=0  gamma_specify=off  gamma_priority=High  gamma=0  rho_specify=off  rho_priority=High  rho=0 kg/m^3  Xc_specify=off  Xc_priority=High  Xc=0  X_specify=off  X_priority=High  X=0  Y_specify=off  Y_priority=High  Y=0  CV_specify=off  CV_priority=High  CV=0
  FCV22 : simCryogenics_lib/Elements/Valve  CVmax=1.5  ControlInputMin=0  ControlInputMax=100  Xt=0.86  Rv=100  lin_v=0  lim_v=0  K=2.4e-5 m^1.50000*kg^0.50000/s/bar^0.50000  Cmd_specify=off  Cmd_priority=High  Cmd=0  gamma_specify=off  gamma_priority=High  gamma=0  rho_specify=off  rho_priority=High  rho=0 kg/m^3  Xc_specify=off  Xc_priority=High  Xc=0  X_specify=off  X_priority=High  X=0  Y_specify=off  Y_priority=High  Y=0  CV_specify=off  CV_priority=High  CV=0
  FT61 : simCryogenics_lib/Sensors/FT
  FT62 : Scope
  FT63 : Scope
  FT64 : simCryogenics_lib/Sensors/FT
  FT65 : simCryogenics_lib/Sensors/FT
  FT66 : Scope
  Gain11 : Gain  Gain=-10
  M src31 : simCryogenics_lib/Sources_Sinks/M src  M=0 kg/s
  M src32 : simCryogenics_lib/Sources_Sinks/M src  M=0 kg/s
  M src33 : simCryogenics_lib/Sources_Sinks/M src  M=0 kg/s
  Mixer19 : simCryogenics_lib/Elements/Mixer2
  Mux28 : Mux  Inputs=2
  Mux29 : Mux  Inputs=2
  Mux30 : Mux  Inputs=2
  P/T src21 : simCryogenics_lib/Sources_Sinks/P//T src  P=1.2 bar  T=4.4 K
  P/T src22 : simCryogenics_lib/Sources_Sinks/P//T src  P=1.2 bar  T=4.4 K
  PS-Simulink Converter{111..121} (11 alike) : nesl_utility/PS-Simulink Converter  PhysicalDomain=network_engine_domain  SubClassName=ps_output  LeftPortType=input  RightPortType=output  PseudoPeriodic=off  Frequencies=[]  Unit=1  AffineConversion=off
  PhaseSep11 : simCryogenics_lib/Elements/PhaseSep  Ideal1=1  DeltaT1=0.05 K  N1=10  h1=400 W/K  Ideal2=1  DeltaT2=0.05 K  N2=10  h2=400 W/K  hmax=0.870 m  S=0.0402 m^2  P0=1.25 bar  h0=50  T0=4.5 K
  Simulink-PS Converter{41..44} (4 alike) : nesl_utility/Simulink-PS Converter  PhysicalDomain=network_engine_domain  SubClassName=ps_input  LeftPortType=input  RightPortType=output  PseudoPeriodic=off  Frequencies=[]  NoiseDistribution=none  NoiseParameters=[]  Unit=1  AffineConversion=off  InputFiltering=off  SimscapeFilterOrder=1  InputFilterTimeConstant=0.001  UdotUserProvided=1
  TT41 : Scope
  TT42 : Scope
  TT43 : simCryogenics_lib/Sensors/PTT
  TT44 : Scope
  scope31 : Scope
  scope32 : Scope
  scope33 : Scope
  to_coldbox : PMIOPort  Port=1  Side=Left
  from_dewar : PMIOPort  Port=2  Side=Right
  wires:
  Bias22/1 -> scope32/1, Simulink-PS Converter43/1
  PS-Simulink Converter113/1 -> Mux30/2
  PS-Simulink Converter119/1 -> Mux29/2
  Mux30/1 -> TT42/1
  Mux29/1 -> TT44/1
  PS-Simulink Converter118/1 -> Mux28/1
  PS-Simulink Converter112/1 -> Mux30/1
  PS-Simulink Converter115/1 -> FT62/1
  PS-Simulink Converter120/1 -> scope33/1, Bias21/1
  PS-Simulink Converter111/1 -> FT66/1
  Gain11/1 -> Bias22/1
  PS-Simulink Converter114/1 -> Mux28/2
  PS-Simulink Converter116/1 -> Mux29/1
  Constant32/1 -> Simulink-PS Converter44/1
  Constant31/1 -> Simulink-PS Converter42/1
  Mux28/1 -> TT41/1
  Bias21/1 -> Gain11/1
  PS-Simulink Converter121/1 -> scope31/1
  Constant30/1 -> Simulink-PS Converter41/1
  PS-Simulink Converter117/1 -> FT63/1
  connections:
  FCV00 2 11/LConn2 -- Distributor17/RConn1
  Simulink-PS Converter41/RConn1 -- PhaseSep11/RConn4
  PS-Simulink Converter115/LConn1 -- FT61/RConn1
  PS-Simulink Converter117/LConn1 -- FT65/RConn1
  BP_out-E21/RConn1 -- PS-Simulink Converter113/LConn1
  BP_out-E22/RConn1 -- PS-Simulink Converter119/LConn1
  BP_out-E22/RConn2 -- PS-Simulink Converter116/LConn1
  FT61/LConn1 -- TT43/LConn1 -- FCV00 2 11/RConn1 -- Mixer19/LConn1
  FCV21/RConn1 -- Mixer19/LConn2 -- FT64/LConn1 -- BP_out-E22/LConn1
  PhaseSep11/LConn2 -- P/T src21/RConn1
  Distributor17/RConn2 -- FCV21/LConn2
  Simulink-PS Converter42/RConn1 -- FCV00 2 11/LConn1
  P/T src22/RConn1 -- PhaseSep11/LConn3
  PhaseSep11/RConn2 -- M src32/RConn1
  from_dewar/RConn1 -- Distributor17/LConn1
  FCV22/LConn2 -- PhaseSep11/LConn1 -- BP_out-E21/LConn1 -- FT65/LConn1
  FCV22/LConn1 -- Simulink-PS Converter44/RConn1
  PS-Simulink Converter121/LConn1 -- PhaseSep11/LConn5
  PhaseSep11/LConn4 -- Mixer19/RConn1
  M src33/RConn1 -- PhaseSep11/RConn3
  M src31/RConn1 -- PhaseSep11/RConn1
  TT43/RConn1 -- PS-Simulink Converter118/LConn1
  PS-Simulink Converter111/LConn1 -- FT64/RConn1
  Simulink-PS Converter43/RConn1 -- FCV21/LConn1
  FCV22/RConn1 -- to_coldbox/RConn1
  TT43/RConn2 -- PS-Simulink Converter114/LConn1
  BP_out-E21/RConn2 -- PS-Simulink Converter112/LConn1
  PS-Simulink Converter120/LConn1 -- PhaseSep11/RConn5

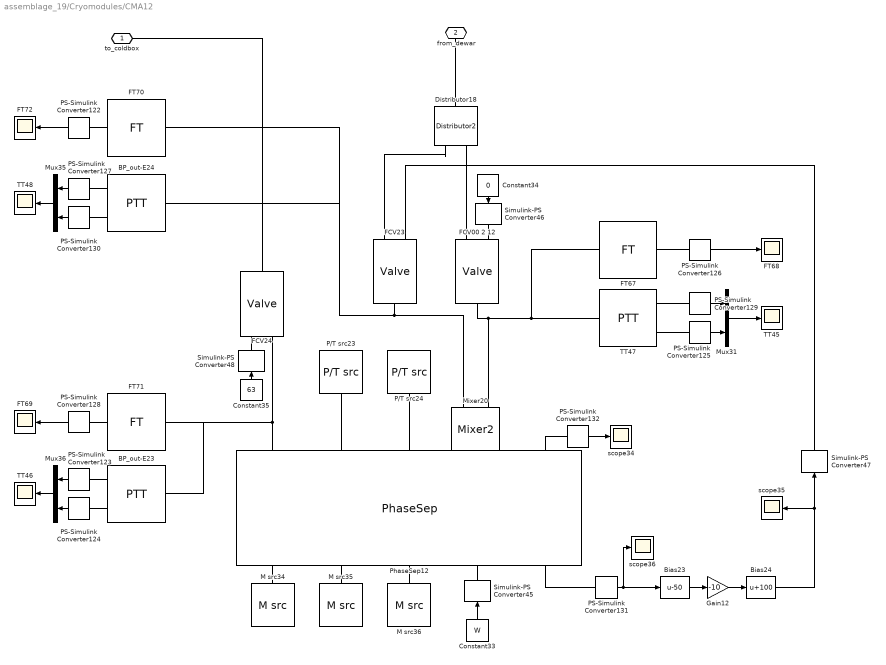
== system assemblage_19/Cryomodules/CMA12 ==
  BP_out-E23 : simCryogenics_lib/Sensors/PTT
  BP_out-E24 : simCryogenics_lib/Sensors/PTT
  Bias23 : Bias  Bias=-50
  Bias24 : Bias  Bias=100
  Constant33 : Constant  Value=W
  Constant34 : Constant  Value=0
  Constant35 : Constant  Value=63
  Distributor18 : simCryogenics_lib/Elements/Distributor2
  FCV00 2 12 : simCryogenics_lib/Elements/Valve  CVmax=0.2  ControlInputMin=0  ControlInputMax=100  Xt=0.86  Rv=100  lin_v=0  lim_v=0  K=2.4e-5 m^1.50000*kg^0.50000/s/bar^0.50000  Cmd_specify=off  Cmd_priority=High  Cmd=0  gamma_specify=off  gamma_priority=High  gamma=0  rho_specify=off  rho_priority=High  rho=0 kg/m^3  Xc_specify=off  Xc_priority=High  Xc=0  X_specify=off  X_priority=High  X=0  Y_specify=off  Y_priority=High  Y=0  CV_specify=off  CV_priority=High  CV=0
  FCV23 : simCryogenics_lib/Elements/Valve  CVmax=1.25  ControlInputMin=0  ControlInputMax=100  Xt=0.86  Rv=150  lin_v=0  lim_v=0  K=2.4e-5 m^1.50000*kg^0.50000/s/bar^0.50000  Cmd_specify=off  Cmd_priority=High  Cmd=0  gamma_specify=off  gamma_priority=High  gamma=0  rho_specify=off  rho_priority=High  rho=0 kg/m^3  Xc_specify=off  Xc_priority=High  Xc=0  X_specify=off  X_priority=High  X=0  Y_specify=off  Y_priority=High  Y=0  CV_specify=off  CV_priority=High  CV=0
  FCV24 : simCryogenics_lib/Elements/Valve  CVmax=1.5  ControlInputMin=0  ControlInputMax=100  Xt=0.86  Rv=100  lin_v=0  lim_v=0  K=2.4e-5 m^1.50000*kg^0.50000/s/bar^0.50000  Cmd_specify=off  Cmd_priority=High  Cmd=0  gamma_specify=off  gamma_priority=High  gamma=0  rho_specify=off  rho_priority=High  rho=0 kg/m^3  Xc_specify=off  Xc_priority=High  Xc=0  X_specify=off  X_priority=High  X=0  Y_specify=off  Y_priority=High  Y=0  CV_specify=off  CV_priority=High  CV=0
  FT67 : simCryogenics_lib/Sensors/FT
  FT68 : Scope
  FT69 : Scope
  FT70 : simCryogenics_lib/Sensors/FT
  FT71 : simCryogenics_lib/Sensors/FT
  FT72 : Scope
  Gain12 : Gain  Gain=-10
  M src34 : simCryogenics_lib/Sources_Sinks/M src  M=0 kg/s
  M src35 : simCryogenics_lib/Sources_Sinks/M src  M=0 kg/s
  M src36 : simCryogenics_lib/Sources_Sinks/M src  M=0 kg/s
  Mixer20 : simCryogenics_lib/Elements/Mixer2
  Mux31 : Mux  Inputs=2
  Mux35 : Mux  Inputs=2
  Mux36 : Mux  Inputs=2
  P/T src23 : simCryogenics_lib/Sources_Sinks/P//T src  P=1.2 bar  T=4.4 K
  P/T src24 : simCryogenics_lib/Sources_Sinks/P//T src  P=1.2 bar  T=4.4 K
  PS-Simulink Converter{122..132} (11 alike) : nesl_utility/PS-Simulink Converter  PhysicalDomain=network_engine_domain  SubClassName=ps_output  LeftPortType=input  RightPortType=output  PseudoPeriodic=off  Frequencies=[]  Unit=1  AffineConversion=off
  PhaseSep12 : simCryogenics_lib/Elements/PhaseSep  Ideal1=1  DeltaT1=0.05 K  N1=10  h1=400 W/K  Ideal2=1  DeltaT2=0.05 K  N2=10  h2=400 W/K  hmax=0.870 m  S=0.0402 m^2  P0=1.25 bar  h0=50  T0=4.5 K
  Simulink-PS Converter{45..48} (4 alike) : nesl_utility/Simulink-PS Converter  PhysicalDomain=network_engine_domain  SubClassName=ps_input  LeftPortType=input  RightPortType=output  PseudoPeriodic=off  Frequencies=[]  NoiseDistribution=none  NoiseParameters=[]  Unit=1  AffineConversion=off  InputFiltering=off  SimscapeFilterOrder=1  InputFilterTimeConstant=0.001  UdotUserProvided=1
  TT45 : Scope
  TT46 : Scope
  TT47 : simCryogenics_lib/Sensors/PTT
  TT48 : Scope
  scope34 : Scope
  scope35 : Scope
  scope36 : Scope
  to_coldbox : PMIOPort  Port=1  Side=Left
  from_dewar : PMIOPort  Port=2  Side=Right
  wires:
  PS-Simulink Converter126/1 -> FT68/1
  PS-Simulink Converter129/1 -> Mux31/1
  Bias23/1 -> Gain12/1
  Constant35/1 -> Simulink-PS Converter48/1
  Gain12/1 -> Bias24/1
  Constant34/1 -> Simulink-PS Converter46/1
  Mux36/1 -> TT46/1
  PS-Simulink Converter124/1 -> Mux36/2
  PS-Simulink Converter125/1 -> Mux31/2
  Mux35/1 -> TT48/1
  PS-Simulink Converter132/1 -> scope34/1
  PS-Simulink Converter127/1 -> Mux35/1
  PS-Simulink Converter128/1 -> FT69/1
  Bias24/1 -> scope35/1, Simulink-PS Converter47/1
  Constant33/1 -> Simulink-PS Converter45/1
  PS-Simulink Converter122/1 -> FT72/1
  PS-Simulink Converter123/1 -> Mux36/1
  PS-Simulink Converter130/1 -> Mux35/2
  Mux31/1 -> TT45/1
  PS-Simulink Converter131/1 -> scope36/1, Bias23/1
  connections:
  FCV24/LConn2 -- PhaseSep12/LConn1 -- BP_out-E23/LConn1 -- FT71/LConn1
  PhaseSep12/RConn2 -- M src35/RConn1
  PhaseSep12/LConn2 -- P/T src23/RConn1
  FCV00 2 12/LConn2 -- Distributor18/RConn1
  Simulink-PS Converter46/RConn1 -- FCV00 2 12/LConn1
  TT47/RConn2 -- PS-Simulink Converter125/LConn1
  FCV23/RConn1 -- Mixer20/LConn2 -- FT70/LConn1 -- BP_out-E24/LConn1
  P/T src24/RConn1 -- PhaseSep12/LConn3
  FT67/LConn1 -- TT47/LConn1 -- FCV00 2 12/RConn1 -- Mixer20/LConn1
  FCV24/LConn1 -- Simulink-PS Converter48/RConn1
  BP_out-E24/RConn2 -- PS-Simulink Converter127/LConn1
  PS-Simulink Converter126/LConn1 -- FT67/RConn1
  Distributor18/RConn2 -- FCV23/LConn2
  Simulink-PS Converter47/RConn1 -- FCV23/LConn1
  BP_out-E23/RConn1 -- PS-Simulink Converter124/LConn1
  from_dewar/RConn1 -- Distributor18/LConn1
  PS-Simulink Converter132/LConn1 -- PhaseSep12/LConn5
  BP_out-E24/RConn1 -- PS-Simulink Converter130/LConn1
  PS-Simulink Converter128/LConn1 -- FT71/RConn1
  M src34/RConn1 -- PhaseSep12/RConn1
  PhaseSep12/LConn4 -- Mixer20/RConn1
  FCV24/RConn1 -- to_coldbox/RConn1
  M src36/RConn1 -- PhaseSep12/RConn3
  Simulink-PS Converter45/RConn1 -- PhaseSep12/RConn4
  PS-Simulink Converter131/LConn1 -- PhaseSep12/RConn5
  PS-Simulink Converter122/LConn1 -- FT70/RConn1
  TT47/RConn1 -- PS-Simulink Converter129/LConn1
  BP_out-E23/RConn2 -- PS-Simulink Converter123/LConn1
